simulink model "AGTF30SysSS_PExPIn"  (R2021b)
settings: Solver=FixedStepDiscrete  StartTime=0.0  StopTime=0; %MWS.In.Ts  FixedStep=1  RelTol=1e-3  EnableMultiTasking=on
values from neighbouring files (symbols this model uses):
  MWS = setup_initialize(MWS,startPt,SSsolverSP)    [Setup_Simulation.m]    (also in run_AGTF30e_script.m = Setup_Simulation(inputMethod,MWS.In,filename,Mdl,SSsolverSP,)
libraries: simulink x66, Lib_Solve_SSNRSolverJC_TMATS x1
(part 2 of 2)

== system AGTF30SysSS_PExPIn/DepFormat/Primary Set-Point/LPCRline Max Error Term ==
  EngIndep : Inport
  Compare To Constant1 : simulink/Logic and Bit Operations/Compare To Constant  relop=~=  const=21  OutDataTypeStr=boolean
  Compare To Zero : simulink/Logic and Bit Operations/Compare To Zero  relop=>  OutDataTypeStr=boolean
      link override Compare: Operator=>  OutDataTypeStr=boolean
  Constant : Constant  Value=MWS.Init.Solver.Limits.LPCRL_Max
  Constant1 : Constant  Value=MWS.Init.Solver.Targets.Opt
  Demux : Demux  Outputs=[5 1 1]
  Logical Operator : Logic  AllPortsSameDT=off  OutDataTypeStr=boolean
  Sum1 : Sum  Inputs=|+-
  Terminator : Terminator
  Terminator1 : Terminator
  Er : Outport
  LimVio : Outport  Port=2
  wires:
  Demux/3 -> Terminator1/1
  Demux/1 -> Terminator/1
  Sum1/1 -> Compare To Zero/1, Er/1
  EngIndep/1 -> Demux/1
  Demux/2 -> Sum1/1
  Constant/1 -> Sum1/2
  Constant1/1 -> Compare To Constant1/1
  Compare To Constant1/1 -> Logical Operator/1
  Compare To Zero/1 -> Logical Operator/2
  Logical Operator/1 -> LimVio/1

== system AGTF30SysSS_PExPIn/DepFormat/Primary Set-Point/LPCRline Min Error Term ==
  EngIndep : Inport
  Compare To Constant1 : simulink/Logic and Bit Operations/Compare To Constant  relop=~=  const=20  OutDataTypeStr=boolean
  Compare To Zero : simulink/Logic and Bit Operations/Compare To Zero  relop=<  OutDataTypeStr=boolean
      link override Compare: Operator=<  OutDataTypeStr=boolean
  Constant : Constant  Value=MWS.Init.Solver.Limits.LPCRL_Min
  Constant1 : Constant  Value=MWS.Init.Solver.Targets.Opt
  Demux : Demux  Outputs=[5 1 1]
  Logical Operator : Logic  AllPortsSameDT=off  OutDataTypeStr=boolean
  Sum1 : Sum  Inputs=|+-
  Terminator : Terminator
  Terminator1 : Terminator
  Er : Outport
  LimVio : Outport  Port=2
  wires:
  Logical Operator/1 -> LimVio/1
  Compare To Zero/1 -> Logical Operator/2
  Compare To Constant1/1 -> Logical Operator/1
  Constant1/1 -> Compare To Constant1/1
  Constant/1 -> Sum1/2
  Demux/2 -> Sum1/1
  EngIndep/1 -> Demux/1
  Sum1/1 -> Er/1, Compare To Zero/1
  Demux/1 -> Terminator/1
  Demux/3 -> Terminator1/1

== system AGTF30SysSS_PExPIn/DepFormat/Primary Set-Point/LPCSM Min Error Term ==
  EngBus : Inport
  Bus Selector : BusSelector  OutputSignals=SM.SMLPC
  Compare To Constant1 : simulink/Logic and Bit Operations/Compare To Constant  relop=~=  const=12  OutDataTypeStr=boolean
  Compare To Zero : simulink/Logic and Bit Operations/Compare To Zero  relop=<  OutDataTypeStr=boolean
      link override Compare: Operator=<  OutDataTypeStr=boolean
  Constant : Constant  Value=MWS.Init.Solver.Limits.LPCSM_Min
  Constant1 : Constant  Value=MWS.Init.Solver.Targets.Opt
  Logical Operator : Logic  AllPortsSameDT=off  OutDataTypeStr=boolean
  Sum1 : Sum  Inputs=|+-
  Er : Outport
  LimVio : Outport  Port=2
  wires:
  Sum1/1 -> Compare To Zero/1, Er/1
  EngBus/1 -> Bus Selector/1
  Bus Selector/1 -> Sum1/1  "<SMLPC>"
  Constant/1 -> Sum1/2
  Constant1/1 -> Compare To Constant1/1
  Compare To Constant1/1 -> Logical Operator/1
  Compare To Zero/1 -> Logical Operator/2
  Logical Operator/1 -> LimVio/1

== system AGTF30SysSS_PExPIn/DepFormat/Primary Set-Point/LPTNcMap Max Error Term ==
  EngBus : Inport
  Bus Selector : BusSelector  OutputSignals=Data.LPT_Data.NcMap
  Compare To Constant1 : simulink/Logic and Bit Operations/Compare To Constant  relop=~=  const=31  OutDataTypeStr=boolean
  Compare To Zero : simulink/Logic and Bit Operations/Compare To Zero  relop=>  OutDataTypeStr=boolean
      link override Compare: Operator=>  OutDataTypeStr=boolean
  Constant : Constant  Value=MWS.Init.Solver.Limits.LPTNcMap_Max
  Constant1 : Constant  Value=MWS.Init.Solver.Targets.Opt
  Logical Operator : Logic  AllPortsSameDT=off  OutDataTypeStr=boolean
  Sum1 : Sum  Inputs=|+-
  Er : Outport
  LimVio : Outport  Port=2
  wires:
  Logical Operator/1 -> LimVio/1
  Compare To Zero/1 -> Logical Operator/2
  Compare To Constant1/1 -> Logical Operator/1
  Constant1/1 -> Compare To Constant1/1
  Constant/1 -> Sum1/2
  Bus Selector/1 -> Sum1/1  "<NcMap>"
  EngBus/1 -> Bus Selector/1
  Sum1/1 -> Er/1, Compare To Zero/1

== system AGTF30SysSS_PExPIn/DepFormat/Primary Set-Point/LPTNcMap Min Error Term ==
  EngBus : Inport
  Bus Selector : BusSelector  OutputSignals=Data.LPT_Data.NcMap
  Compare To Constant1 : simulink/Logic and Bit Operations/Compare To Constant  relop=~=  const=30  OutDataTypeStr=boolean
  Compare To Zero : simulink/Logic and Bit Operations/Compare To Zero  relop=<  OutDataTypeStr=boolean
      link override Compare: Operator=<  OutDataTypeStr=boolean
  Constant : Constant  Value=MWS.Init.Solver.Limits.LPTNcMap_Min
  Constant1 : Constant  Value=MWS.Init.Solver.Targets.Opt
  Logical Operator : Logic  AllPortsSameDT=off  OutDataTypeStr=boolean
  Sum1 : Sum  Inputs=|+-
  Er : Outport
  LimVio : Outport  Port=2
  wires:
  Sum1/1 -> Compare To Zero/1, Er/1
  EngBus/1 -> Bus Selector/1
  Bus Selector/1 -> Sum1/1  "<NcMap>"
  Constant/1 -> Sum1/2
  Constant1/1 -> Compare To Constant1/1
  Compare To Constant1/1 -> Logical Operator/1
  Compare To Zero/1 -> Logical Operator/2
  Logical Operator/1 -> LimVio/1

== system AGTF30SysSS_PExPIn/DepFormat/Primary Set-Point/LPTPRMap Max Error Term ==
  EngBus : Inport
  Bus Selector : BusSelector  OutputSignals=Data.LPT_Data.PRMap
  Compare To Constant1 : simulink/Logic and Bit Operations/Compare To Constant  relop=~=  const=33  OutDataTypeStr=boolean
  Compare To Zero : simulink/Logic and Bit Operations/Compare To Zero  relop=>  OutDataTypeStr=boolean
      link override Compare: Operator=>  OutDataTypeStr=boolean
  Constant : Constant  Value=MWS.Init.Solver.Limits.LPTPRMap_Max
  Constant1 : Constant  Value=MWS.Init.Solver.Targets.Opt
  Logical Operator : Logic  AllPortsSameDT=off  OutDataTypeStr=boolean
  Sum1 : Sum  Inputs=|+-
  Er : Outport
  LimVio : Outport  Port=2
  wires:
  Sum1/1 -> Compare To Zero/1, Er/1
  EngBus/1 -> Bus Selector/1
  Bus Selector/1 -> Sum1/1  "<PRMap>"
  Constant/1 -> Sum1/2
  Constant1/1 -> Compare To Constant1/1
  Compare To Constant1/1 -> Logical Operator/1
  Compare To Zero/1 -> Logical Operator/2
  Logical Operator/1 -> LimVio/1

== system AGTF30SysSS_PExPIn/DepFormat/Primary Set-Point/LPTPRMap Min Error Term ==
  EngBus : Inport
  Bus Selector : BusSelector  OutputSignals=Data.LPT_Data.PRMap
  Compare To Constant1 : simulink/Logic and Bit Operations/Compare To Constant  relop=~=  const=32  OutDataTypeStr=boolean
  Compare To Zero : simulink/Logic and Bit Operations/Compare To Zero  relop=<  OutDataTypeStr=boolean
      link override Compare: Operator=<  OutDataTypeStr=boolean
  Constant : Constant  Value=MWS.Init.Solver.Limits.LPTPRMap_Min
  Constant1 : Constant  Value=MWS.Init.Solver.Targets.Opt
  Logical Operator : Logic  AllPortsSameDT=off  OutDataTypeStr=boolean
  Sum1 : Sum  Inputs=|+-
  Er : Outport
  LimVio : Outport  Port=2
  wires:
  Logical Operator/1 -> LimVio/1
  Compare To Zero/1 -> Logical Operator/2
  Compare To Constant1/1 -> Logical Operator/1
  Constant1/1 -> Compare To Constant1/1
  Constant/1 -> Sum1/2
  Bus Selector/1 -> Sum1/1  "<PRMap>"
  EngBus/1 -> Bus Selector/1
  Sum1/1 -> Er/1, Compare To Zero/1

== system AGTF30SysSS_PExPIn/DepFormat/Primary Set-Point/N1 Max Error Term ==
  EngBus : Inport
  Bus Selector : BusSelector  OutputSignals=Shaft.N_Fan
  Compare To Constant1 : simulink/Logic and Bit Operations/Compare To Constant  relop=~=  const=8  OutDataTypeStr=boolean
  Compare To Zero : simulink/Logic and Bit Operations/Compare To Zero  relop=>  OutDataTypeStr=boolean
      link override Compare: Operator=>  OutDataTypeStr=boolean
  Constant : Constant  Value=MWS.Init.Solver.Limits.N1_Max
  Constant1 : Constant  Value=MWS.Init.Solver.Targets.Opt
  Logical Operator : Logic  AllPortsSameDT=off  OutDataTypeStr=boolean
  Sum1 : Sum  Inputs=|+-
  Er : Outport
  LimVio : Outport  Port=2
  wires:
  Sum1/1 -> Compare To Zero/1, Er/1
  EngBus/1 -> Bus Selector/1
  Bus Selector/1 -> Sum1/1  "<N_Fan>"
  Constant/1 -> Sum1/2
  Constant1/1 -> Compare To Constant1/1
  Compare To Constant1/1 -> Logical Operator/1
  Compare To Zero/1 -> Logical Operator/2
  Logical Operator/1 -> LimVio/1

== system AGTF30SysSS_PExPIn/DepFormat/Primary Set-Point/N3 Max Error Term ==
  EngBus : Inport
  Bus Selector : BusSelector  OutputSignals=Shaft.N_HPC
  Compare To Constant1 : simulink/Logic and Bit Operations/Compare To Constant  relop=~=  const=9  OutDataTypeStr=boolean
  Compare To Zero : simulink/Logic and Bit Operations/Compare To Zero  relop=>  OutDataTypeStr=boolean
      link override Compare: Operator=>  OutDataTypeStr=boolean
  Constant : Constant  Value=MWS.Init.Solver.Limits.N3_Max
  Constant1 : Constant  Value=MWS.Init.Solver.Targets.Opt
  Logical Operator : Logic  AllPortsSameDT=off  OutDataTypeStr=boolean
  Sum1 : Sum  Inputs=|+-
  Er : Outport
  LimVio : Outport  Port=2
  wires:
  Logical Operator/1 -> LimVio/1
  Compare To Zero/1 -> Logical Operator/2
  Compare To Constant1/1 -> Logical Operator/1
  Constant1/1 -> Compare To Constant1/1
  Constant/1 -> Sum1/2
  Bus Selector/1 -> Sum1/1  "<N_HPC>"
  EngBus/1 -> Bus Selector/1
  Sum1/1 -> Er/1, Compare To Zero/1

== system AGTF30SysSS_PExPIn/DepFormat/Primary Set-Point/Ps3 Max Error Term ==
  EngBus : Inport
  Bus Selector : BusSelector  OutputSignals=S36.Ps
  Compare To Constant1 : simulink/Logic and Bit Operations/Compare To Constant  relop=~=  const=7  OutDataTypeStr=boolean
  Compare To Zero : simulink/Logic and Bit Operations/Compare To Zero  relop=>  OutDataTypeStr=boolean
      link override Compare: Operator=>  OutDataTypeStr=boolean
  Constant : Constant  Value=MWS.Init.Solver.Limits.Ps3_Max
  Constant1 : Constant  Value=MWS.Init.Solver.Targets.Opt
  Logical Operator : Logic  AllPortsSameDT=off  OutDataTypeStr=boolean
  Sum1 : Sum  Inputs=|+-
  Er : Outport
  LimVio : Outport  Port=2
  wires:
  Logical Operator/1 -> LimVio/1
  Compare To Zero/1 -> Logical Operator/2
  Compare To Constant1/1 -> Logical Operator/1
  Constant1/1 -> Compare To Constant1/1
  Constant/1 -> Sum1/2
  Bus Selector/1 -> Sum1/1  "<Ps>"
  EngBus/1 -> Bus Selector/1
  Sum1/1 -> Er/1, Compare To Zero/1

== system AGTF30SysSS_PExPIn/DepFormat/Primary Set-Point/T3 Max Error Term ==
  EngBus : Inport
  Bus Selector : BusSelector  OutputSignals=S36.Tt
  Compare To Constant1 : simulink/Logic and Bit Operations/Compare To Constant  relop=~=  const=5  OutDataTypeStr=boolean
  Compare To Zero : simulink/Logic and Bit Operations/Compare To Zero  relop=>  OutDataTypeStr=boolean
      link override Compare: Operator=>  OutDataTypeStr=boolean
  Constant : Constant  Value=MWS.Init.Solver.Limits.T3_Max
  Constant1 : Constant  Value=MWS.Init.Solver.Targets.Opt
  Logical Operator : Logic  AllPortsSameDT=off  OutDataTypeStr=boolean
  Sum1 : Sum  Inputs=|+-
  Er : Outport
  LimVio : Outport  Port=2
  wires:
  Constant/1 -> Sum1/2
  Bus Selector/1 -> Sum1/1  "<Tt>"
  EngBus/1 -> Bus Selector/1
  Sum1/1 -> Er/1, Compare To Zero/1
  Compare To Constant1/1 -> Logical Operator/1
  Logical Operator/1 -> LimVio/1
  Compare To Zero/1 -> Logical Operator/2
  Constant1/1 -> Compare To Constant1/1

== system AGTF30SysSS_PExPIn/DepFormat/Primary Set-Point/T4 Error Term ==
  EngBus : Inport
  Bus Selector : BusSelector  OutputSignals=S4.Tt
  Constant : Constant  Value=MWS.Init.Solver.Targets.T4
  Sum1 : Sum  Inputs=|+-
  T4Er : Outport
  wires:
  Sum1/1 -> T4Er/1  "T4Er"
  EngBus/1 -> Bus Selector/1
  Bus Selector/1 -> Sum1/1  "<Tt>"
  Constant/1 -> Sum1/2

== system AGTF30SysSS_PExPIn/DepFormat/Primary Set-Point/T4 Max Error Term ==
  EngBus : Inport
  Bus Selector : BusSelector  OutputSignals=S4.Tt
  Compare To Constant1 : simulink/Logic and Bit Operations/Compare To Constant  relop=~=  const=6  OutDataTypeStr=boolean
  Compare To Zero : simulink/Logic and Bit Operations/Compare To Zero  relop=>  OutDataTypeStr=boolean
      link override Compare: Operator=>  OutDataTypeStr=boolean
  Constant : Constant  Value=MWS.Init.Solver.Limits.T4_Max
  Constant1 : Constant  Value=MWS.Init.Solver.Targets.Opt
  Logical Operator : Logic  AllPortsSameDT=off  OutDataTypeStr=boolean
  Sum1 : Sum  Inputs=|+-
  Er : Outport
  LimVio : Outport  Port=2
  wires:
  Sum1/1 -> Compare To Zero/1, Er/1
  EngBus/1 -> Bus Selector/1
  Bus Selector/1 -> Sum1/1  "<Tt>"
  Constant/1 -> Sum1/2
  Constant1/1 -> Compare To Constant1/1
  Compare To Constant1/1 -> Logical Operator/1
  Compare To Zero/1 -> Logical Operator/2
  Logical Operator/1 -> LimVio/1

== system AGTF30SysSS_PExPIn/DepFormat/Primary Set-Point/Thrust Error Term ==
  EngBus : Inport
  Bus Selector : BusSelector  OutputSignals=Perf.Fnet
  Nc1 Set Point : Constant  Value=MWS.Init.Solver.Targets.Fn
  Sum1 : Sum  Inputs=|+-
  FnEr : Outport
  wires:
  Nc1 Set Point/1 -> Sum1/2
  Bus Selector/1 -> Sum1/1  "<Fnet>"
  EngBus/1 -> Bus Selector/1
  Sum1/1 -> FnEr/1  "NcEr"

== system AGTF30SysSS_PExPIn/DepFormat/VAFN Set-Point/VAFN FanRL Error Term ==
  EngBus : Inport
  EngIndep : Inport  Port=2
  1-D Lookup Table : Lookup_n-D  NumberOfTableDimensions=1  BreakpointsForDimension1=MWS.Init.Solver.SS.VAFNOpt_NcVec  Table=MWS.Init.Solver.SS.VAFNOpt_RLVec  InternalRulePriority=Speed  RndMeth=Simplest  InputSameDT=on
  Bus Selector : BusSelector  OutputSignals=Data.FAN_Data.NcMap
  Demux : Demux  Outputs=[3 1 3]
  Sum : Sum  Inputs=|+-
  Terminator : Terminator
  Terminator1 : Terminator
  Fan RLine : Outport
  wires:
  EngBus/1 -> Bus Selector/1
  Demux/3 -> Terminator1/1
  Demux/1 -> Terminator/1
  1-D Lookup Table/1 -> Sum/1
  Demux/2 -> Sum/2
  EngIndep/1 -> Demux/1
  Sum/1 -> Fan RLine/1  "Fan RLine"
  Bus Selector/1 -> 1-D Lookup Table/1  "<NcMap>"

== system AGTF30SysSS_PExPIn/DepFormat/VAFN Set-Point/VAFN Max Error Term ==
  InputBus : Inport
  Bus Selector : BusSelector  OutputSignals=VAFN
  Compare To Constant : simulink/Logic and Bit Operations/Compare To Constant  relop=~=  const=3  OutDataTypeStr=boolean
      link override Compare: Operator=~=  OutDataTypeStr=boolean
  Compare To Zero : simulink/Logic and Bit Operations/Compare To Zero  relop=>  OutDataTypeStr=boolean
      link override Compare: Operator=>  OutDataTypeStr=boolean
  Constant : Constant  Value=MWS.Init.Solver.Limits.VAFN_Max
  Constant1 : Constant  Value=MWS.Init.Solver.SS.VAFNOpt
  Logical Operator : Logic  AllPortsSameDT=off  OutDataTypeStr=boolean
  Sum1 : Sum  Inputs=|+-
  Er : Outport
  LimVio : Outport  Port=2
  wires:
  Sum1/1 -> Compare To Zero/1, Er/1
  InputBus/1 -> Bus Selector/1
  Bus Selector/1 -> Sum1/1  "<VAFN>"
  Constant/1 -> Sum1/2
  Constant1/1 -> Compare To Constant/1
  Compare To Constant/1 -> Logical Operator/1
  Compare To Zero/1 -> Logical Operator/2
  Logical Operator/1 -> LimVio/1

== system AGTF30SysSS_PExPIn/DepFormat/VAFN Set-Point/VAFN Min Error Term ==
  InputBus : Inport
  Bus Selector : BusSelector  OutputSignals=VAFN
  Compare To Constant : simulink/Logic and Bit Operations/Compare To Constant  relop=~=  const=2  OutDataTypeStr=boolean
      link override Compare: Operator=~=  OutDataTypeStr=boolean
  Compare To Zero : simulink/Logic and Bit Operations/Compare To Zero  relop=<  OutDataTypeStr=boolean
      link override Compare: Operator=<  OutDataTypeStr=boolean
  Constant : Constant  Value=MWS.Init.Solver.Limits.VAFN_Min
  Constant1 : Constant  Value=MWS.Init.Solver.SS.VAFNOpt
  Logical Operator : Logic  AllPortsSameDT=off  OutDataTypeStr=boolean
  Sum1 : Sum  Inputs=|+-
  Er : Outport
  LimVio : Outport  Port=2
  wires:
  Logical Operator/1 -> LimVio/1
  Compare To Zero/1 -> Logical Operator/2
  Compare To Constant/1 -> Logical Operator/1
  Constant1/1 -> Compare To Constant/1
  Constant/1 -> Sum1/2
  Bus Selector/1 -> Sum1/1  "<VAFN>"
  InputBus/1 -> Bus Selector/1
  Sum1/1 -> Er/1, Compare To Zero/1

== system AGTF30SysSS_PExPIn/DepFormat/VAFN Set-Point/VAFN Sched Error Term ==
  EngBus : Inport
  InputBus : Inport  Port=2
  Bus Selector2 : BusSelector  OutputSignals=VAFN
  Constant : Constant  Value=0
  Sum : Sum  Inputs=|+-
  Terminator : Terminator
  Terminator1 : Terminator
  VAFNEr : Outport
  wires:
  Bus Selector2/1 -> Sum/2  "<VAFN>"
  InputBus/1 -> Terminator1/1, Bus Selector2/1
  Sum/1 -> VAFNEr/1  "VAFN_Er"
  Constant/1 -> Sum/1
  EngBus/1 -> Terminator/1

== system AGTF30SysSS_PExPIn/DepFormat/VBV Set-Point/VBV Max Error Term ==
  InputBus : Inport
  Bus Selector : BusSelector  OutputSignals=VBV
  Compare To Constant : simulink/Logic and Bit Operations/Compare To Constant  relop=~=  const=3  OutDataTypeStr=boolean
      link override Compare: Operator=~=  OutDataTypeStr=boolean
  Compare To Zero : simulink/Logic and Bit Operations/Compare To Zero  relop=>  OutDataTypeStr=boolean
      link override Compare: Operator=>  OutDataTypeStr=boolean
  Constant : Constant  Value=MWS.Init.Solver.Limits.VBV_Max
  Constant1 : Constant  Value=MWS.Init.Solver.SS.VBVOpt
  Logical Operator : Logic  AllPortsSameDT=off  OutDataTypeStr=boolean
  Sum1 : Sum  Inputs=|+-
  Er : Outport
  LimVio : Outport  Port=2
  wires:
  Sum1/1 -> Compare To Zero/1, Er/1
  InputBus/1 -> Bus Selector/1
  Bus Selector/1 -> Sum1/1  "<VBV>"
  Constant/1 -> Sum1/2
  Constant1/1 -> Compare To Constant/1
  Compare To Constant/1 -> Logical Operator/1
  Compare To Zero/1 -> Logical Operator/2
  Logical Operator/1 -> LimVio/1

== system AGTF30SysSS_PExPIn/DepFormat/VBV Set-Point/VBV Min Error Term ==
  InputBus : Inport
  Bus Selector : BusSelector  OutputSignals=VBV
  Compare To Constant : simulink/Logic and Bit Operations/Compare To Constant  relop=~=  const=2  OutDataTypeStr=boolean
      link override Compare: Operator=~=  OutDataTypeStr=boolean
  Compare To Zero : simulink/Logic and Bit Operations/Compare To Zero  relop=<  OutDataTypeStr=boolean
      link override Compare: Operator=<  OutDataTypeStr=boolean
  Constant : Constant  Value=MWS.Init.Solver.Limits.VBV_Min
  Constant1 : Constant  Value=MWS.Init.Solver.SS.VBVOpt
  Logical Operator : Logic  AllPortsSameDT=off  OutDataTypeStr=boolean
  Sum1 : Sum  Inputs=|+-
  Er : Outport
  LimVio : Outport  Port=2
  wires:
  Logical Operator/1 -> LimVio/1
  Compare To Zero/1 -> Logical Operator/2
  Compare To Constant/1 -> Logical Operator/1
  Constant1/1 -> Compare To Constant/1
  Constant/1 -> Sum1/2
  Bus Selector/1 -> Sum1/1  "<VBV>"
  InputBus/1 -> Bus Selector/1
  Sum1/1 -> Er/1, Compare To Zero/1

== system AGTF30SysSS_PExPIn/DepFormat/VBV Set-Point/VBV Sched Error Term ==
  EngBus : Inport
  InputBus : Inport  Port=2
  Bus Selector2 : BusSelector  OutputSignals=VBV
  Constant : Constant  Value=0
  Sum : Sum  Inputs=|+-
  Terminator : Terminator
  Terminator1 : Terminator
  VBVEr : Outport
  wires:
  Constant/1 -> Sum/1
  Sum/1 -> VBVEr/1  "VBV_Er"
  Bus Selector2/1 -> Sum/2  "<VBV>"
  EngBus/1 -> Terminator/1
  InputBus/1 -> Terminator1/1, Bus Selector2/1

== system AGTF30SysSS_PExPIn/DepFormat/Primary Set-Point/Corrected Fan Speed Error Term/Nc1 Sched Error Term ==
  EngBus : Inport
  InputBus : Inport  Port=2
  Bus Selector2 : BusSelector  OutputSignals=Data.FAN_Data.Nc
  Constant : Constant  Value=0
  Sum : Sum  Inputs=|+-
  Terminator : Terminator
  Terminator1 : Terminator
  Nc1Er : Outport
  wires:
  Constant/1 -> Sum/1
  Sum/1 -> Nc1Er/1  "Nc1_Er"
  EngBus/1 -> Bus Selector2/1, Terminator/1
  InputBus/1 -> Terminator1/1
  Bus Selector2/1 -> Sum/2  "<Nc>"
